simulink model "tuberia"  (R2016a)
settings: Solver=ode4  StartTime=0.0  StopTime=12  FixedStep=0.05  RelTol=1e-3
settings Model: Creator=omar  LastModifiedBy=omar

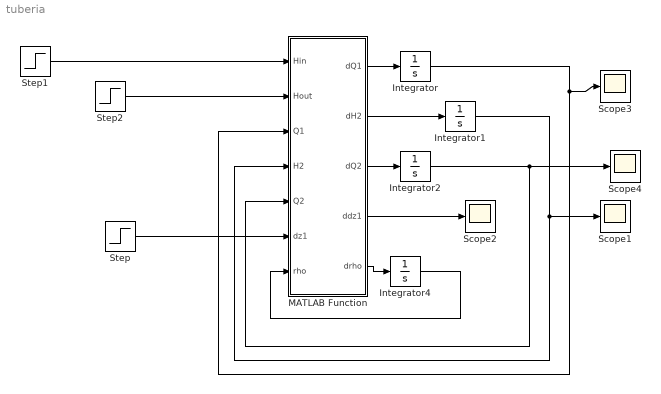
== system tuberia ==
  Integrator : Integrator  InitialCondition=4.25e-3
  Integrator1 : Integrator  InitialCondition=5
  Integrator2 : Integrator  InitialCondition=4.25e-3
  Integrator4 : Integrator  InitialCondition=7e-5
  MATLAB Function : MATLAB Function  TreatAsAtomicUnit=on
  Scope{1..4} (4 alike) : Scope
  Step : Step  Time=5  After=20  SampleTime=0
  Step1 : Step  Time=5  Before=6.4  After=6  SampleTime=0
  Step2 : Step  Time=5  Before=3.6  After=3.4  SampleTime=0
  wires:
  MATLAB Function/1(dQ1) -> Integrator/1
  MATLAB Function/2(dH2) -> Integrator1/1
  MATLAB Function/3(dQ2) -> Integrator2/1
  MATLAB Function/5(drho) -> Integrator4/1
  Integrator4/1 -> MATLAB Function/7(rho)
  Integrator2/1 -> Scope4/1, MATLAB Function/5(Q2)
  Integrator1/1 -> Scope1/1, MATLAB Function/4(H2)
  Integrator/1 -> Scope3/1, MATLAB Function/3(Q1)
  Step/1 -> MATLAB Function/6(dz1)
  Step1/1 -> MATLAB Function/1(Hin)
  Step2/1 -> MATLAB Function/2(Hout)
  MATLAB Function/4(ddz1) -> Scope2/1

== matlab function tuberia/MATLAB Function ==
  data: Hin input; dQ1 output; Hout input; Q1 input; H2 input; Q2 input; dz1 input; rho input; dH2 output; dQ2 output; ddz1 output; drho output
function [dQ1,dH2,dQ2,ddz1,drho] = fcn(Hin,Hout,Q1,H2,Q2,dz1,rho)


L=85;%%%68.147
D=6.35e-2;%%%6.271e-2
b=407.75;
% tau=1.72e-2;
tau=1;
g=9.81;
A=pi*(D/2)^2;
% A=pi*((1*2.54)/2)^2;
muu=tau/(2*D*A);
f=0.0226;
    
    if(dz1==0)
        dH2=0;
        dQ1=0;
        dQ2=0;
    else
        dQ1=-((g*A)/dz1)*(H2-Hin)-f*muu*Q1*abs(Q1);
        dH2=-((b^2)/(g*A*dz1))*(Q2-Q1+rho*(H2)^0.5);
        dQ2=-((g*A)/(L-dz1))*(Hout-H2)-f*muu*Q2*abs(Q2);
    end
    
    ddz1=0;
    drho=0;
